simulink model "Basics_1"  (R2015a)
settings: Solver=ode4  StartTime=0.0  StopTime=10.0  FixedStep=1e-4  RelTol=1e-3
settings Model: Creator=ayyrao  LastModifiedBy=ayyrao

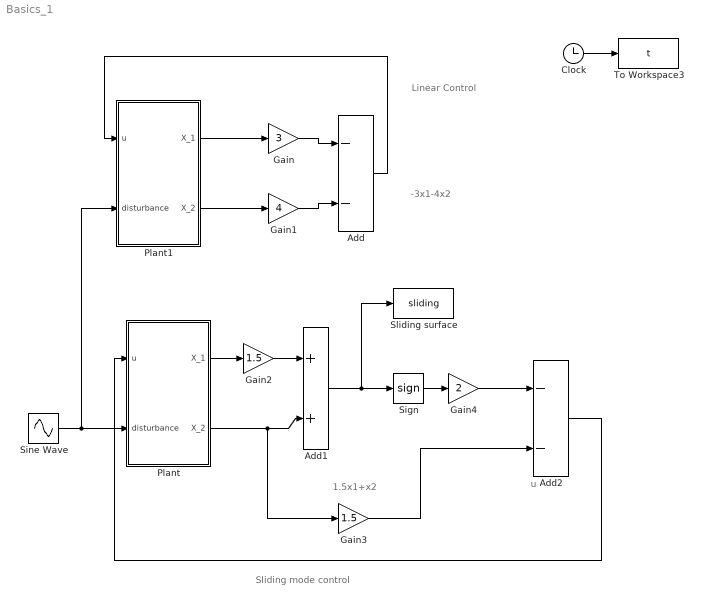
== system Basics_1 ==
  note: Sliding mode control
  note: Linear Control
  note: u
  note: 1.5x1+x2
  note: -3x1-4x2
  Add : Sum  Inputs=--
  Add1 : Sum
  Add2 : Sum  Inputs=--
  Clock : Clock
  Gain : Gain  Gain=3
  Gain1 : Gain  Gain=4
  Gain2 : Gain  Gain=1.5
  Gain3 : Gain  Gain=1.5
  Gain4 : Gain  Gain=2
  Plant : Subsystem
  Plant1 : Subsystem
  Sign : Signum
  Sine Wave : Sin  Frequency=2  SampleTime=0
  Sliding surface : ToWorkspace  VariableName=sliding  SampleTime=-1
  To Workspace3 : ToWorkspace  VariableName=t  SampleTime=-1
  wires:
  Plant1/2(X_2) -> Gain1/1
  Plant1/1(X_1) -> Gain/1
  Gain/1 -> Add/1
  Gain1/1 -> Add/2
  Add/1 -> Plant1/1(u)
  Clock/1 -> To Workspace3/1
  Sine Wave/1 -> Plant1/2(disturbance), Plant/2(disturbance)
  Plant/1(X_1) -> Gain2/1
  Gain2/1 -> Add1/1
  Plant/2(X_2) -> Gain3/1, Add1/2
  Add1/1 -> Sign/1, Sliding surface/1
  Gain3/1 -> Add2/2
  Add2/1 -> Plant/1(u)
  Sign/1 -> Gain4/1
  Gain4/1 -> Add2/1

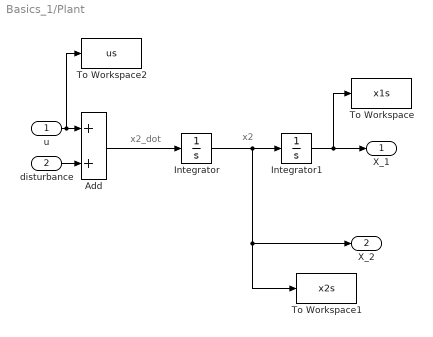
== system Basics_1/Plant ==
  note: x2_dot
  note: x2
  u : Inport
  disturbance : Inport  Port=2
  Add : Sum
  Integrator : Integrator  InitialCondition=-2
  Integrator1 : Integrator  InitialCondition=1
  To Workspace : ToWorkspace  VariableName=x1s  SampleTime=-1
  To Workspace1 : ToWorkspace  VariableName=x2s  SampleTime=-1
  To Workspace2 : ToWorkspace  VariableName=us  SampleTime=-1
  X_1 : Outport
  X_2 : Outport  Port=2
  wires:
  Integrator/1 -> Integrator1/1, X_2/1, To Workspace1/1
  Integrator1/1 -> X_1/1, To Workspace/1
  u/1 -> Add/1, To Workspace2/1
  disturbance/1 -> Add/2
  Add/1 -> Integrator/1

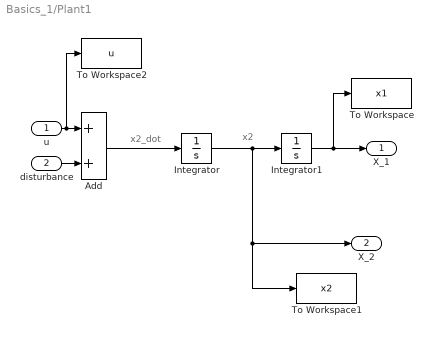
== system Basics_1/Plant1 ==
  note: x2
  note: x2_dot
  u : Inport
  disturbance : Inport  Port=2
  Add : Sum
  Integrator : Integrator  InitialCondition=-2
  Integrator1 : Integrator  InitialCondition=1
  To Workspace : ToWorkspace  VariableName=x1  SampleTime=-1
  To Workspace1 : ToWorkspace  VariableName=x2  SampleTime=-1
  To Workspace2 : ToWorkspace  VariableName=u  SampleTime=-1
  X_1 : Outport
  X_2 : Outport  Port=2
  wires:
  Add/1 -> Integrator/1
  disturbance/1 -> Add/2
  u/1 -> To Workspace2/1, Add/1
  Integrator1/1 -> To Workspace/1, X_1/1
  Integrator/1 -> To Workspace1/1, X_2/1, Integrator1/1
